simulink model "DroneSimulation"  (R2019a)
settings: Solver=ode23s  StartTime=0.0  StopTime=100  FixedStep=.01  RelTol=1e-5  AbsTol=1e-5
libraries: simulink x1
settings Model: Creator=hp  LastModifiedBy=hp
settings DataIOCC: SaveState=on

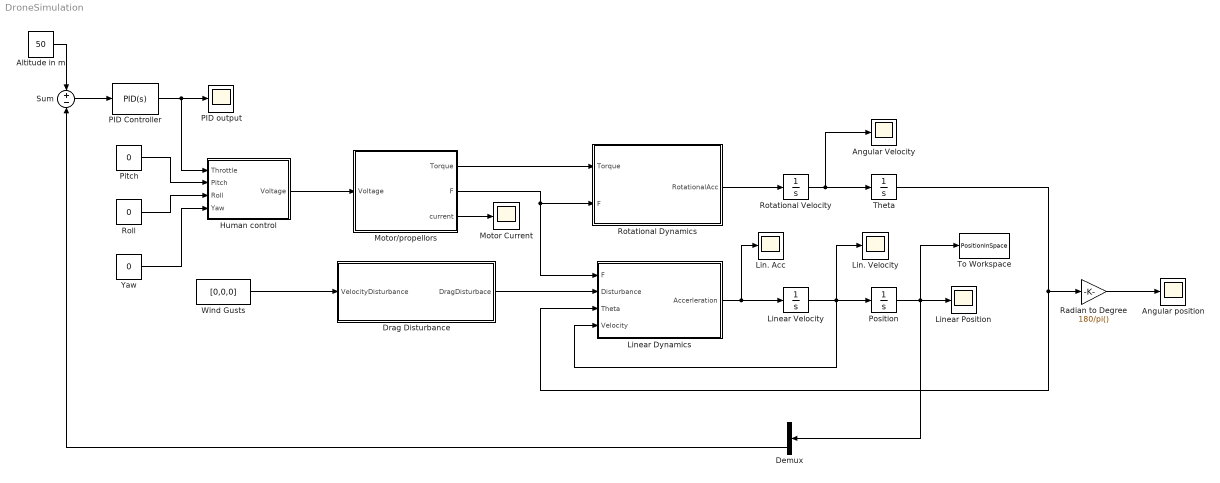
== system DroneSimulation ==
  Altitude in m : Constant  Value=50
  Angular Velocity : Scope
  Angular position : Scope
  Demux : Demux  Outputs=3
  Drag Disturbance : MATLAB Function  TreatAsAtomicUnit=on
  Human control : MATLAB Function  TreatAsAtomicUnit=on
  "Lin. Acc " : Scope
  Lin. Velocity : Scope
  Linear Dynamics : MATLAB Function  TreatAsAtomicUnit=on
  Linear Position : Scope
  Linear Velocity : Integrator
  Motor Current : Scope
  Motor/propellors : MATLAB Function  TreatAsAtomicUnit=on
  PID Controller : simulink/Continuous/PID Controller  Controller=PID  Form=Parallel  TimeDomain=Continuous-time  SampleTime=-1  IntegratorMethod=Forward Euler  FilterMethod=Forward Euler  ControllerParametersSource=internal  P=9  I=.5  D=10  UseFilter=on  N=100  TunerSelectOption=Transfer Function Based (PID Tuner App)  InitialConditionSource=internal  InitialConditionForIntegrator=1  InitialConditionForFilter=0  DifferentiatorICPrevScaledInput=0  ExternalReset=none  TrackingMode=off  Kt=1  LimitOutput=on  UpperSaturationLimit=100  LowerSaturationLimit=0  LinearizeAsGain=on  AntiWindupMode=clamping  Kb=1  POutMin=[]  POutMax=[]  IOutMin=[]  IOutMax=[]  DOutMin=[]  DOutMax=[]  NOutMin=[]  NOutMax=[]  SumOutMin=[]  SumOutMax=[]  SaturationOutMin=[]  SaturationOutMax=[]  PParamMin=[]  PParamMax=[]  IParamMin=[]  IParamMax=[]  DParamMin=[]  DParamMax=[]  NParamMin=[]  NParamMax=[]  KbParamMin=[]  KbParamMax=[]  KtParamMin=[]  KtParamMax=[]  KbOutMin=[]  KbOutMax=[]  KtOutMin=[]  KtOutMax=[]  IntegratorOutMin=[]  IntegratorOutMax=[]  FilterOutMin=[]  FilterOutMax=[]  SumI1OutMin=[]  SumI1OutMax=[]  SumI2OutMin=[]  SumI2OutMax=[]  SumI3OutMin=[]  SumI3OutMax=[]  SumI4OutMin=[]  SumI4OutMax=[]  SumDOutMin=[]  SumDOutMax=[]  DifferentiatorOutMin=[]  DifferentiatorOutMax=[]  FilterDiffOutCoefMin=[]  FilterDiffOutCoefMax=[]  ReciprocalOutMin=[]  ReciprocalOutMax=[]  SumDenOutMin=[]  SumDenOutMax=[]  SumNumOutMin=[]  SumNumOutMax=[]  DivideOutMin=[]  DivideOutMax=[]  IntegratorContinuousStateAttributes=''  IntegratorStateMustResolveToSignalObject=off  IntegratorRTWStateStorageClass=Auto  FilterContinuousStateAttributes=''  FilterStateMustResolveToSignalObject=off  FilterRTWStateStorageClass=Auto  ParallelPVariant=InternalParameters  IdealPVariant=Disabled  IVariant=InternalParameters  DVariant=InternalParameters  IntegratorVariant=Continuous  SatVariant=Enabled  AWVariant=ContClampingParallel  PCopyVariant=Disabled  TRVariant=Disabled  FdbkBlocksVariant=Forward  IdealPFdbkVariant=Disabled  SatFdbkVariant=Disabled  DerivativeFilterVariant=ContFilter  NVariant=InternalParameters  NCopyVariant=Disabled  FilterICVariant=InternalICsFilter  IntegratorICVariant=InternalICs  ExternalResetVariant=Disabled  TRSumVariant=Passthrough  SumFdbkVariant=Disabled  SumVariant=Sum_PID
  PID output : Scope
  Pitch : Constant  Value=0
  Position : Integrator
  Radian to Degree : Gain  Gain=180/pi()
  Roll : Constant  Value=0
  "Rotational Dynamics " : MATLAB Function  TreatAsAtomicUnit=on
  Rotational Velocity : Integrator
  Sum : Sum  Inputs=+-
  Theta : Integrator
  To Workspace : ToWorkspace  VariableName=PositionInSpace  SampleTime=-1
      settings: Save2DSignal=2-D array (concatenate along first dimension)
  Wind Gusts : Constant  Value=[0,0,0]
  Yaw : Constant  Value=0
  wires:
  Motor/propellors/1(Torque) -> "Rotational Dynamics "/1(Torque)
  "Rotational Dynamics "/1(RotationalAcc) -> Rotational Velocity/1
  Motor/propellors/2(F) -> Linear Dynamics/1(F), "Rotational Dynamics "/2(F)
  Theta/1 -> Radian to Degree/1, Linear Dynamics/3(Theta)
  Linear Dynamics/1(Accerleration) -> "Lin. Acc "/1, Linear Velocity/1
  Linear Velocity/1 -> Lin. Velocity/1, Linear Dynamics/4(Velocity), Position/1
  Drag Disturbance/1(DragDisturbace) -> Linear Dynamics/2(Disturbance)
  Wind Gusts/1 -> Drag Disturbance/1(VelocityDisturbance)
  Human control/1(Voltage) -> Motor/propellors/1(Voltage)
  Pitch/1 -> Human control/2(Pitch)
  Roll/1 -> Human control/3(Roll)
  Yaw/1 -> Human control/4(Yaw)
  Rotational Velocity/1 -> Theta/1, Angular Velocity/1
  Position/1 -> Demux/1, To Workspace/1, Linear Position/1
  Motor/propellors/3(current) -> Motor Current/1
  Radian to Degree/1 -> Angular position/1
  PID Controller/1 -> PID output/1, Human control/1(Throttle)
  Demux/3 -> Sum/2
  Altitude in m/1 -> Sum/1
  Sum/1 -> PID Controller/1

== matlab function DroneSimulation/Rotational Dynamics  ==
  data: Torque input; RotationalAcc output; F input
function RotationalAcc = fcn( Torque , F)
Moment = [0 0 0];
RotationalAcc = [0 0 0];
Inertia = [0.003 0.003 0.007];
Moment(1) = ((F(3)+F(4))*(.237/2)   -  ((F(1)+F(2))*(.237/2)));
Moment(2) = ((F(3)+F(2))*(.237/2)   -  ((F(1)+F(4))*(.237/2)));
Moment(3) = Torque(4) - Torque(1) + Torque(2) - Torque(3);

for i = 1:3
     RotationalAcc(i) = Moment(i)/Inertia(i) ;
end

end

== matlab function DroneSimulation/Motor//propellors ==
  data: Voltage input; Torque output; F output; current output
function [Torque,F,current] = fcn(Voltage)

RPM = [0 0 0 0];Torque = [0 0 0 0];F = [0 0 0 0];current = [0 0 0 0];
for i=1:4
RPM(i) = -2.6931*(power(Voltage(i),3))   +  1400* Voltage(i);
ct = (2*(power(10,-15))*(power(RPM(i),3)))+   (4*(power(10,-11))*(power(RPM(i),2)))+(3*(power(10,-7))*(RPM(i)))+.1013;
F(i) = ct * 1.225 * power((RPM(i)/60),2) * power(.2,4);
Torque(i) = (4*(power(10,-14))*(power(RPM(i),3))) +  (8*(power(10,-12))*(power(RPM(i),2)))  +  (3*(power(10,-6))*(RPM(i)));
current(i) = Torque(i) * 1400;
end

end

== matlab function DroneSimulation/Linear Dynamics ==
  data: F input; Accerleration output; Disturbance input; Theta input; Velocity input
function Accerleration = fcn(F, Disturbance, Theta, Velocity)
% function Accerleration = fcn( F, Disturbance , Theta, Velocity)

m = .743;
cd = 1;
A= [0.0197 0.0197 .0512];
g= 9.81;
rho = 1.225;

Accerleration = [0 0 0];Force= [0 0 0]; Fprop = [0 0 0 ];

Fprop(1) = (F(1)+F(2)+F(3)+F(4))*sin(Theta(2)) * cos(Theta(1)); 
Fprop(2) = (F(1)+F(2)+F(3)+F(4))*sin(Theta(1)) * cos(Theta(2));
Fprop(3) = (F(1)+F(2)+F(3)+F(4))*cos(Theta(2)) * cos(Theta(1));
if (Fprop(1)&&Fprop(2))~=0
ThetaXY = -atan(Fprop(1)/Fprop(2));
XY2D = sqrt( Fprop(1)^2  +  Fprop(2)^2);

if Fprop(3)>=0
    Fprop(1) = XY2D * sin(ThetaXY + Theta(3));
    Fprop(2) = XY2D * cos(ThetaXY + Theta(3));
else
    Fprop(1) = XY2D * sin(ThetaXY - Theta(3));
    Fprop(2) = XY2D * cos(ThetaXY - Theta(3));
end
end
if Velocity(1)<=0
   Force(1) = Fprop(1) - Disturbance(1) + (.5*rho*power(Velocity(1),2)*A(1)* cd); 
else
   Force(1) = Fprop(1) - Disturbance(1) - (.5*rho*power(Velocity(1),2)*A(1)* cd); 
end


if Velocity(2)<=0
   Force(2) = Fprop(2) - Disturbance(2) + (.5*rho*power(Velocity(2),2)*A(2)* cd); 
else
   Force(2) = Fprop(2) - Disturbance(2) - (.5*rho*power(Velocity(2),2)*A(2)* cd); 
end

if Velocity(3)<=0
   Force(3) = Fprop(3) - Disturbance(3) + (.5*rho*power(Velocity(3),2)*A(3)* cd) - (m*g); 
else
   Force(3) = Fprop(3) - Disturbance(3) - (.5*rho*power(Velocity(3),2)*A(3)* cd) - (m*g); 
end

for i=1:3
    Accerleration(i) = Force(i)/m;
end

% end

== matlab function DroneSimulation/Drag Disturbance ==
  data: VelocityDisturbance input; DragDisturbace output
function DragDisturbace = fcn(VelocityDisturbance)
A = [0.0197 0.0197 0.0512];
DragDisturbace = [0 0 0];
rho = 1.225;
cd=1;


for i =1:3
    if VelocityDisturbance(i)<0
        DragDisturbace(i) = 0.5 * rho * VelocityDisturbance(i)^2  * A(i) *cd;
    else
        DragDisturbace(i) = -0.5 * rho * VelocityDisturbance(i)^2  * A(i) *cd;

end


end

== matlab function DroneSimulation/Human control ==
  data: Throttle input; Voltage output; Pitch input; Roll input; Yaw input
function Voltage = fcn(Throttle , Pitch , Roll , Yaw)
c=0;
if (Pitch+Roll+Yaw)/2   >   100 - Throttle
 c = (Pitch+Roll+Yaw)/2 -(100 - Throttle);
end

if (Pitch+Roll+Yaw)/2   >  Throttle
    if   c<  (Pitch+Roll+Yaw)/2   -  Throttle
        c =  (Pitch+Roll+Yaw)/2   -  Throttle;
    end
end

Pitch = Pitch -(c/3)*2;
Roll = Roll -(c/3)*2;
Yaw = Yaw -(c/3)*2;

Voltage = [(Throttle -  (Pitch+Roll+Yaw)/2)*11.4/100 ,(Throttle -  (Pitch-Roll-Yaw)/2)*11.4/100, (Throttle -  (-Pitch-Roll+Yaw)/2)*11.4/100 , (Throttle -  (-Pitch+Roll-Yaw)/2)*11.4/100];
end
